simulink model "simulink_nivastyring"  (R2024b)
settings: Solver=VariableStepAuto  StartTime=0.0  StopTime=1000  RelTol=1e-6
undefined symbols (not defined in the file or in its folder): A_tank1, A_tank2, k, p
settings Model: Creator=serin  LastModifiedBy=seyon
settings SolverCC: ZeroCrossAlgorithm=Adaptive
settings DebuggingCC: IgnoredZcDiagnostic=none

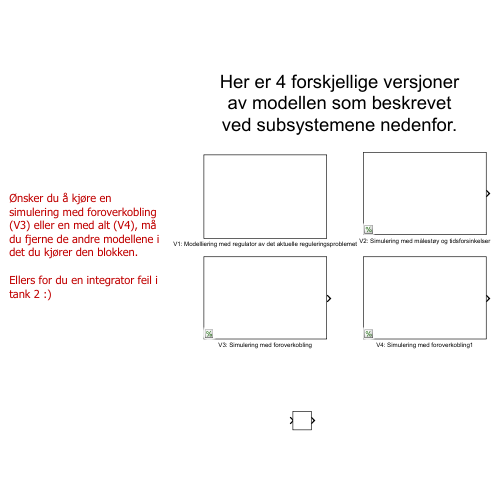
[thumbnail: Simulink's stored preview of the top-level diagram]
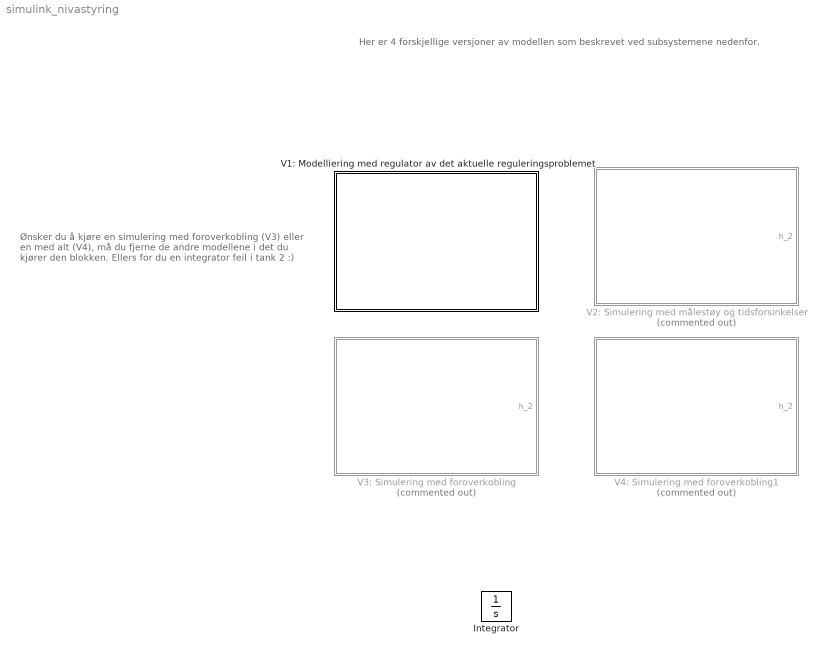
== system simulink_nivastyring ==
  note: Ønsker du å kjøre en simulering med foroverkobling (V3) eller en med alt (V4), må du fjerne de andre modellene i det du kjører den blokken.
      |
      | Ellers for du en integrator feil i tank 2 :)
  note: Her er 4 forskjellige versjoner av modellen som beskrevet ved subsystemene nedenfor.
  Integrator : Integrator
  V1: Modelliering med regulator av det aktuelle reguleringsproblemet : Subsystem
  V2: Simulering med målestøy og tidsforsinkelser : Subsystem  Commented=on
  V3: Simulering med foroverkobling : Subsystem  Commented=on
  V4: Simulering med foroverkobling1 : Subsystem  Commented=on

== system simulink_nivastyring/V1: Modelliering med regulator av det aktuelle reguleringsproblemet ==
  Scope : Scope  NumInputPorts=4
  Subsystem1 : Subsystem
  Subsystem2 : Subsystem
  Subsystem3 : Subsystem
  Subsystem4 : Subsystem
  wires:
  Subsystem1/1(h1) -> Scope/4  "tau = 0"
  Subsystem2/1(h1) -> Scope/1  "tau = 3"
  Subsystem3/1(h1) -> Scope/2  "tau = 6"
  Subsystem4/1(h1) -> Scope/3  "tau = 12"

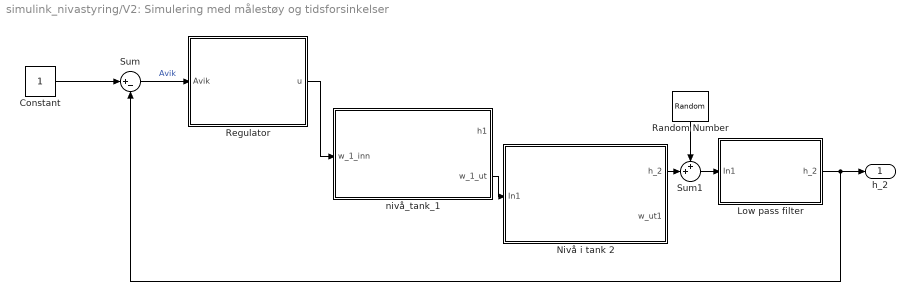
== system simulink_nivastyring/V2: Simulering med målestøy og tidsforsinkelser ==
  Constant : Constant
  Low pass filter : Subsystem
  Nivå i tank 2 : Subsystem
  Random Number : RandomNumber  Variance=0.001  Seed=23  SampleTime=1
  Regulator : Subsystem
  Sum : Sum  Inputs=|+-
  Sum1 : Sum  Inputs=++|
  nivå_tank_1 : Subsystem
  h_2 : Outport
  wires:
  Constant/1 -> Sum/1
  Nivå i tank 2/1(h_2) -> Sum1/2
  Sum1/1 -> Low pass filter/1(In1)
  Random Number/1 -> Sum1/1
  Low pass filter/1(h_2) -> h_2/1, Sum/2
  nivå_tank_1/2(w_1_ut) -> Nivå i tank 2/1(In1)
  Regulator/1(u) -> nivå_tank_1/1(w_1_inn)
  Sum/1 -> Regulator/1(Avik)  "Avik"

== system simulink_nivastyring/V3: Simulering med foroverkobling ==
  Constant : Constant
  Forstyrrelse1 : Subsystem
  Nivå i tank 2 : Subsystem
  Sum : Sum  Inputs=|+-
  Sum1 : Sum  Inputs=|++
  nivå_tank_1 : Subsystem
  regulator : Subsystem
  h_2 : Outport
  wires:
  Constant/1 -> Sum/1
  Nivå i tank 2/1(h_2) -> h_2/1, Sum/2
  nivå_tank_1/2(w_1_ut) -> Nivå i tank 2/1(In1)
  Sum/1 -> regulator/1(Avik)  "Avik"
  regulator/1(u) -> Sum1/1
  Forstyrrelse1/1(Out1) -> Sum1/2
  Sum1/1 -> nivå_tank_1/1(w_1_inn)

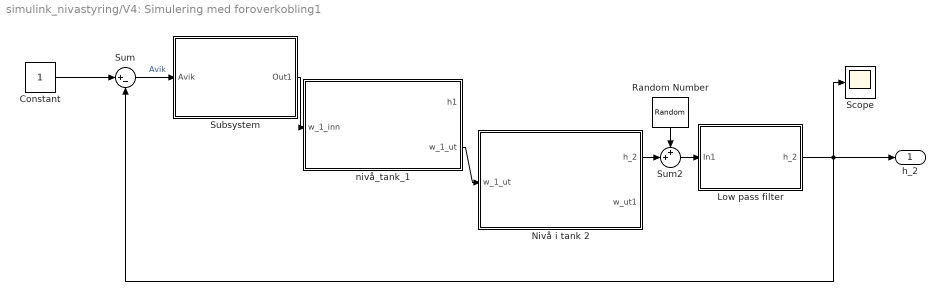
== system simulink_nivastyring/V4: Simulering med foroverkobling1 ==
  Constant : Constant
  Low pass filter : Subsystem
  Nivå i tank 2 : Subsystem
  Random Number : RandomNumber  Variance=0.001  Seed=23  SampleTime=1
  Scope : Scope
  Subsystem : Subsystem
  Sum : Sum  Inputs=|+-
  Sum2 : Sum  Inputs=++|
  nivå_tank_1 : Subsystem
  h_2 : Outport
  wires:
  Constant/1 -> Sum/1
  Nivå i tank 2/1(h_2) -> Sum2/2
  Random Number/1 -> Sum2/1
  nivå_tank_1/2(w_1_ut) -> Nivå i tank 2/1(w_1_ut)
  Sum2/1 -> Low pass filter/1(In1)
  Low pass filter/1(h_2) -> Scope/1, h_2/1, Sum/2
  Sum/1 -> Subsystem/1(Avik)  "Avik"
  Subsystem/1(Out1) -> nivå_tank_1/1(w_1_inn)

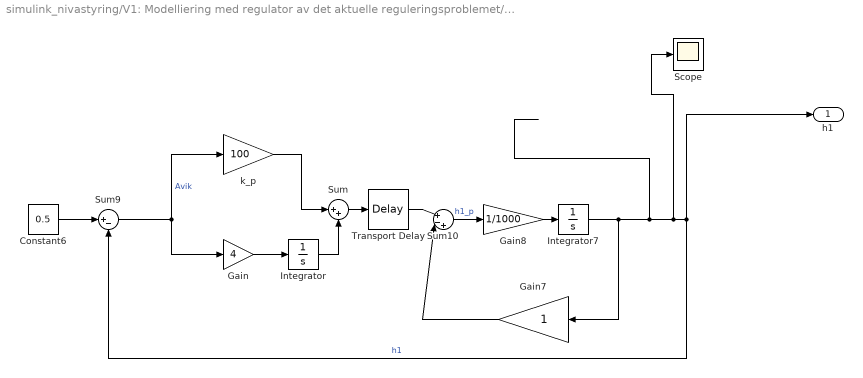
== system simulink_nivastyring/V1: Modelliering med regulator av det aktuelle reguleringsproblemet/Subsystem1 ==
  Constant6 : Constant  Value=0.5
  Gain : Gain  Gain=4
  Gain7 : Gain
  Gain8 : Gain  Gain=1/1000
  Integrator : Integrator
  Integrator7 : Integrator
  Scope : Scope
  Sum : Sum  Inputs=|++
  Sum10 : Sum  Inputs=|+-+
  Sum9 : Sum  Inputs=|+-
  Transport Delay : TransportDelay
  k_p : Gain  Gain=100
  h1 : Outport
  wires:
  Sum9/1 -> Gain/1, k_p/1  "Avik"
  Sum10/1 -> Gain8/1  "h1_p"
  Integrator7/1 -> Scope/1, h1/1, Sum9/2, Gain7/1  "h1"
  Gain7/1 -> Sum10/2
  Gain8/1 -> Integrator7/1
  Constant6/1 -> Sum9/1
  Gain/1 -> Integrator/1
  Integrator/1 -> Sum/2
  k_p/1 -> Sum/1
  Sum/1 -> Transport Delay/1
  Transport Delay/1 -> Sum10/1

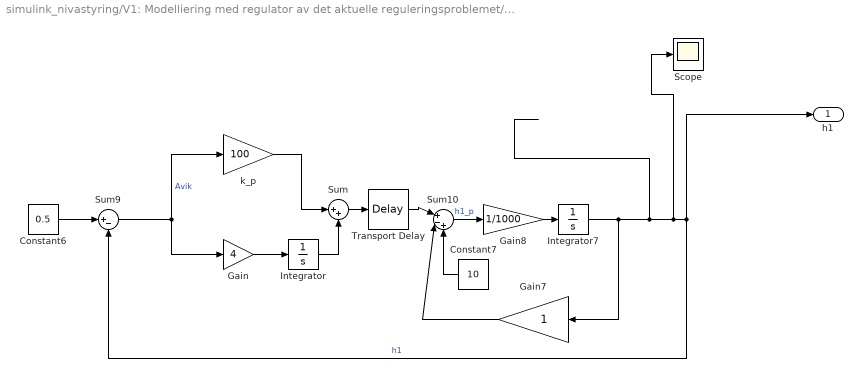
== system simulink_nivastyring/V1: Modelliering med regulator av det aktuelle reguleringsproblemet/Subsystem2 ==
  Constant6 : Constant  Value=0.5
  Constant7 : Constant  Value=10
  Gain : Gain  Gain=4
  Gain7 : Gain
  Gain8 : Gain  Gain=1/1000
  Integrator : Integrator
  Integrator7 : Integrator
  Scope : Scope
  Sum : Sum  Inputs=|++
  Sum10 : Sum  Inputs=|+-+
  Sum9 : Sum  Inputs=|+-
  Transport Delay : TransportDelay
  k_p : Gain  Gain=100
  h1 : Outport
  wires:
  Sum9/1 -> Gain/1, k_p/1  "Avik"
  Sum10/1 -> Gain8/1  "h1_p"
  Integrator7/1 -> Scope/1, h1/1, Sum9/2, Gain7/1  "h1"
  Gain7/1 -> Sum10/2
  Gain8/1 -> Integrator7/1
  Constant6/1 -> Sum9/1
  Constant7/1 -> Sum10/3
  Gain/1 -> Integrator/1
  Integrator/1 -> Sum/2
  k_p/1 -> Sum/1
  Sum/1 -> Transport Delay/1
  Transport Delay/1 -> Sum10/1

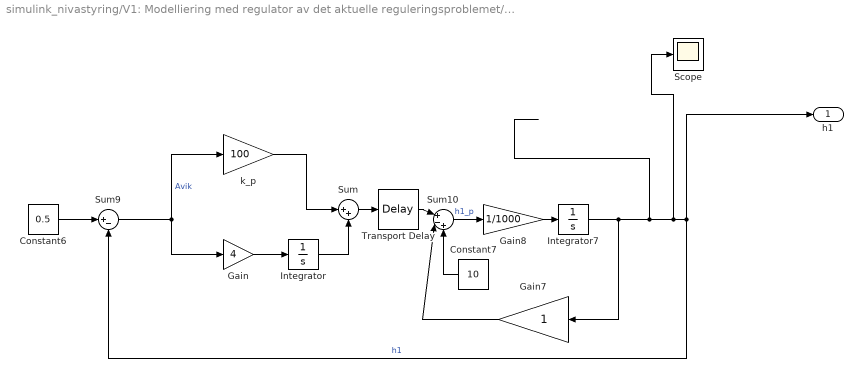
== system simulink_nivastyring/V1: Modelliering med regulator av det aktuelle reguleringsproblemet/Subsystem3 ==
  Constant6 : Constant  Value=0.5
  Constant7 : Constant  Value=10
  Gain : Gain  Gain=4
  Gain7 : Gain
  Gain8 : Gain  Gain=1/1000
  Integrator : Integrator
  Integrator7 : Integrator
  Scope : Scope
  Sum : Sum  Inputs=|++
  Sum10 : Sum  Inputs=|+-+
  Sum9 : Sum  Inputs=|+-
  Transport Delay : TransportDelay  DelayTime=6
  k_p : Gain  Gain=100
  h1 : Outport
  wires:
  Sum9/1 -> Gain/1, k_p/1  "Avik"
  Sum10/1 -> Gain8/1  "h1_p"
  Integrator7/1 -> Scope/1, h1/1, Sum9/2, Gain7/1  "h1"
  Gain7/1 -> Sum10/2
  Gain8/1 -> Integrator7/1
  Constant6/1 -> Sum9/1
  Constant7/1 -> Sum10/3
  Gain/1 -> Integrator/1
  Integrator/1 -> Sum/2
  k_p/1 -> Sum/1
  Sum/1 -> Transport Delay/1
  Transport Delay/1 -> Sum10/1

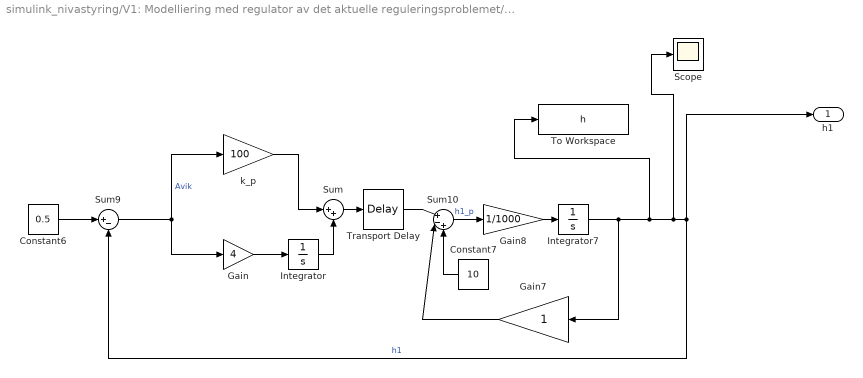
== system simulink_nivastyring/V1: Modelliering med regulator av det aktuelle reguleringsproblemet/Subsystem4 ==
  Constant6 : Constant  Value=0.5
  Constant7 : Constant  Value=10
  Gain : Gain  Gain=4
  Gain7 : Gain
  Gain8 : Gain  Gain=1/1000
  Integrator : Integrator
  Integrator7 : Integrator
  Scope : Scope
  Sum : Sum  Inputs=|++
  Sum10 : Sum  Inputs=|+-+
  Sum9 : Sum  Inputs=|+-
  To Workspace : ToWorkspace  VariableName=h  SaveFormat=Timeseries  SampleTime=-1
  Transport Delay : TransportDelay  DelayTime=12
  k_p : Gain  Gain=100
  h1 : Outport
  wires:
  Sum9/1 -> Gain/1, k_p/1  "Avik"
  Sum10/1 -> Gain8/1  "h1_p"
  Integrator7/1 -> To Workspace/1, Scope/1, h1/1, Sum9/2, Gain7/1  "h1"
  Gain7/1 -> Sum10/2
  Gain8/1 -> Integrator7/1
  Constant6/1 -> Sum9/1
  Constant7/1 -> Sum10/3
  Gain/1 -> Integrator/1
  Integrator/1 -> Sum/2
  k_p/1 -> Sum/1
  Sum/1 -> Transport Delay/1
  Transport Delay/1 -> Sum10/1

== system simulink_nivastyring/V2: Simulering med målestøy og tidsforsinkelser/Low pass filter ==
  In1 : Inport
  Gain : Gain  Gain=0.1
  Integrator : Integrator
  Sum2 : Sum  Inputs=|+-
  h_2 : Outport
  wires:
  Integrator/1 -> h_2/1, Sum2/2
  In1/1 -> Sum2/1
  Sum2/1 -> Gain/1
  Gain/1 -> Integrator/1

== system simulink_nivastyring/V2: Simulering med målestøy og tidsforsinkelser/Nivå i tank 2 ==
  In1 : Inport
  Gain5 : Gain  Gain=k
  Integrator3 : Integrator
  Square Root : Sqrt
  Sum4 : Sum  Inputs=+--
  verdi : Gain  Gain=1/(p*A_tank2)
  h_2 : Outport
  w_ut1 : Outport  Port=2
  wires:
  In1/1 -> Sum4/1
  Sum4/1 -> verdi/1
  Integrator3/1 -> h_2/1, Square Root/1
  Square Root/1 -> Gain5/1
  verdi/1 -> Integrator3/1
  Gain5/1 -> Sum4/2, w_ut1/1  "w_ut"

== system simulink_nivastyring/V2: Simulering med målestøy og tidsforsinkelser/Regulator ==
  Avik : Inport
  regulator : Subsystem  mask{kp=4.5, ki=0.01, wind_up=10}
  u : Outport
  wires:
  regulator/1(w_inn) -> u/1  "u"
  Avik/1 -> regulator/1(In1)

== system simulink_nivastyring/V2: Simulering med målestøy og tidsforsinkelser/nivå_tank_1 ==
  w_1_inn : Inport
  Gain2 : Gain  Gain=k
  Gain3 : Gain  Gain=1/(p*A_tank1)
  Integrator2 : Integrator
  Scope : Scope
  Square Root : Sqrt  OutputSignalType=real
  Sum : Sum  Inputs=|+-
  h1 : Outport
  w_1_ut : Outport  Port=2
  wires:
  Integrator2/1 -> Square Root/1, h1/1  "h1"
  Gain2/1 -> Scope/1, w_1_ut/1, Sum/2
  Sum/1 -> Gain3/1  "h1_p"
  Gain3/1 -> Integrator2/1
  w_1_inn/1 -> Sum/1
  Square Root/1 -> Gain2/1

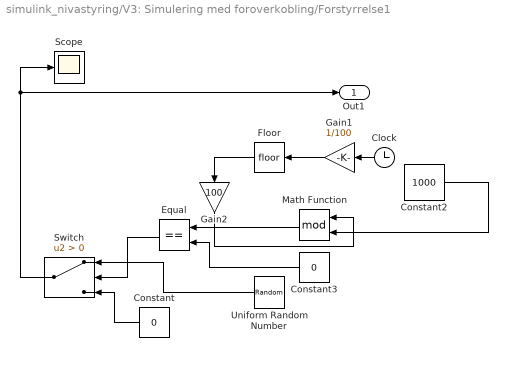
== system simulink_nivastyring/V3: Simulering med foroverkobling/Forstyrrelse1 ==
  Clock : Clock
  Constant : Constant  Value=0
  Constant2 : Constant  Value=1000
  Constant3 : Constant  Value=0
  Equal : RelationalOperator  Operator===  OutDataTypeStr=boolean  RndMeth=Simplest  InputSameDT=off
  Floor : Rounding
  Gain1 : Gain  Gain=1/100
  Gain2 : Gain  Gain=100
  Math Function : Math  Operator=mod
  Scope : Scope
  Switch : Switch  Criteria=u2 > Threshold  SaturateOnIntegerOverflow=off  InputSameDT=off
  Uniform Random Number : UniformRandomNumber  Minimum=0.08  Maximum=0.10  Seed=23  SampleTime=1
  Out1 : Outport
  wires:
  Gain2/1 -> Math Function/1
  Clock/1 -> Gain1/1
  Math Function/1 -> Equal/1
  Switch/1 -> Out1/1, Scope/1
  Constant2/1 -> Math Function/2
  Constant3/1 -> Equal/2
  Gain1/1 -> Floor/1
  Constant/1 -> Switch/3
  Equal/1 -> Switch/2
  Floor/1 -> Gain2/1
  Uniform Random Number/1 -> Switch/1

== system simulink_nivastyring/V3: Simulering med foroverkobling/Nivå i tank 2 ==
  In1 : Inport
  Gain5 : Gain  Gain=k
  Integrator3 : Integrator
  Square Root : Sqrt
  Sum4 : Sum  Inputs=+--
  verdi : Gain  Gain=1/(p*A_tank2)
  h_2 : Outport
  w_ut1 : Outport  Port=2
  wires:
  In1/1 -> Sum4/1
  Sum4/1 -> verdi/1
  Integrator3/1 -> Square Root/1, h_2/1
  Square Root/1 -> Gain5/1
  verdi/1 -> Integrator3/1
  Gain5/1 -> w_ut1/1, Sum4/2  "w_ut"

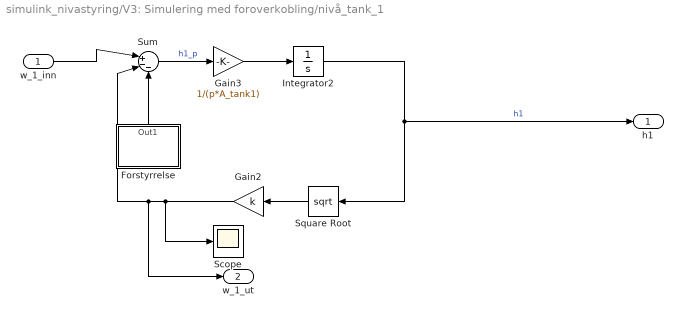
== system simulink_nivastyring/V3: Simulering med foroverkobling/nivå_tank_1 ==
  w_1_inn : Inport
  Forstyrrelse : Subsystem
  Gain2 : Gain  Gain=k
  Gain3 : Gain  Gain=1/(p*A_tank1)
  Integrator2 : Integrator
  Scope : Scope
  Square Root : Sqrt  OutputSignalType=real
  Sum : Sum  Inputs=|+--
  h1 : Outport
  w_1_ut : Outport  Port=2
  wires:
  Integrator2/1 -> Square Root/1, h1/1  "h1"
  Gain2/1 -> Sum/2, w_1_ut/1, Scope/1
  Sum/1 -> Gain3/1  "h1_p"
  Gain3/1 -> Integrator2/1
  w_1_inn/1 -> Sum/1
  Square Root/1 -> Gain2/1
  Forstyrrelse/1(Out1) -> Sum/3

== system simulink_nivastyring/V3: Simulering med foroverkobling/regulator ==
  Avik : Inport
  Rate Limiter : RateLimiter  FallingSlewLimit=-0.01  SampleTimeMode=inherited
  Saturation : Saturate  UpperLimit=4  LowerLimit=0
  ventilen : Subsystem  mask{kp=4.5, ki=0.01, wind_up=10}
  u : Outport
  wires:
  Saturation/1 -> Rate Limiter/1  "u"
  ventilen/1(w_inn) -> Saturation/1
  Avik/1 -> ventilen/1(In1)
  Rate Limiter/1 -> u/1

== system simulink_nivastyring/V4: Simulering med foroverkobling1/Low pass filter ==
  In1 : Inport
  Gain : Gain  Gain=0.1
  Integrator : Integrator
  Sum2 : Sum  Inputs=|+-
  h_2 : Outport
  wires:
  Integrator/1 -> h_2/1, Sum2/2
  In1/1 -> Sum2/1
  Sum2/1 -> Gain/1
  Gain/1 -> Integrator/1

== system simulink_nivastyring/V4: Simulering med foroverkobling1/Nivå i tank 2 ==
  w_1_ut : Inport
  Gain5 : Gain  Gain=k
  Integrator3 : Integrator
  Square Root : Sqrt
  Sum4 : Sum  Inputs=+--
  verdi : Gain  Gain=1/(p*A_tank2)
  h_2 : Outport
  w_ut1 : Outport  Port=2
  wires:
  w_1_ut/1 -> Sum4/1
  Sum4/1 -> verdi/1
  Integrator3/1 -> Square Root/1, h_2/1
  Square Root/1 -> Gain5/1
  verdi/1 -> Integrator3/1
  Gain5/1 -> w_ut1/1, Sum4/2  "w_ut"

== system simulink_nivastyring/V4: Simulering med foroverkobling1/Subsystem ==
  Avik : Inport
  Rate Limiter : RateLimiter  FallingSlewLimit=-0.01  SampleTimeMode=inherited
  Regulator : Subsystem  mask{kp=3, ki=0.0071, wind_up=10}
  Saturation : Saturate  UpperLimit=4  LowerLimit=0
  Sum1 : Sum  Inputs=|++
  Transport Delay : TransportDelay
  forstyrrelse_wv : Subsystem
  Out1 : Outport
  wires:
  Sum1/1 -> Rate Limiter/1  "u"
  Rate Limiter/1 -> Saturation/1
  forstyrrelse_wv/1(Out1) -> Sum1/2
  Transport Delay/1 -> Out1/1
  Regulator/1(w_inn) -> Sum1/1
  Saturation/1 -> Transport Delay/1  "u"
  Avik/1 -> Regulator/1(In1)

== system simulink_nivastyring/V4: Simulering med foroverkobling1/nivå_tank_1 ==
  w_1_inn : Inport
  Forstyrrelse : Subsystem
  Gain2 : Gain  Gain=k
  Gain3 : Gain  Gain=1/(p*A_tank1)
  Integrator2 : Integrator
  Square Root : Sqrt  OutputSignalType=real
  Sum : Sum  Inputs=|+--
  h1 : Outport
  w_1_ut : Outport  Port=2
  wires:
  Integrator2/1 -> Square Root/1, h1/1  "h1"
  Gain2/1 -> w_1_ut/1, Sum/2
  Sum/1 -> Gain3/1  "h1_p"
  Gain3/1 -> Integrator2/1
  w_1_inn/1 -> Sum/1
  Square Root/1 -> Gain2/1
  Forstyrrelse/1(Out1) -> Sum/3

== system simulink_nivastyring/V2: Simulering med målestøy og tidsforsinkelser/Regulator/regulator ==
  In1 : Inport
  Integrator : Integrator
  Rate Limiter : RateLimiter  FallingSlewLimit=-0.01  SampleTimeMode=inherited
  Saturation : Saturate  UpperLimit=4  LowerLimit=0
  Sum1 : Sum  Inputs=|+++
  k_i : Gain  Gain=ki
  k_p : Gain  Gain=kp
  w_inn : Outport
  wires:
  Integrator/1 -> Sum1/1
  In1/1 -> k_p/1, k_i/1
  k_p/1 -> Sum1/2
  Sum1/1 -> Saturation/1
  k_i/1 -> Integrator/1
  Saturation/1 -> Rate Limiter/1  "u"
  Rate Limiter/1 -> w_inn/1

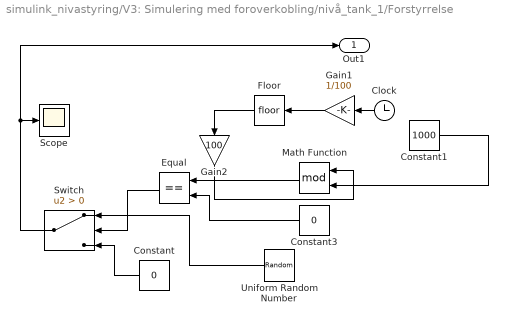
== system simulink_nivastyring/V3: Simulering med foroverkobling/nivå_tank_1/Forstyrrelse ==
  Clock : Clock
  Constant : Constant  Value=0
  Constant1 : Constant  Value=1000
  Constant3 : Constant  Value=0
  Equal : RelationalOperator  Operator===  OutDataTypeStr=boolean  RndMeth=Simplest  InputSameDT=off
  Floor : Rounding
  Gain1 : Gain  Gain=1/100
  Gain2 : Gain  Gain=100
  Math Function : Math  Operator=mod
  Scope : Scope
  Switch : Switch  Criteria=u2 > Threshold  SaturateOnIntegerOverflow=off  InputSameDT=off
  Uniform Random Number : UniformRandomNumber  Minimum=0.08  Maximum=0.10  Seed=23  SampleTime=1
  Out1 : Outport
  wires:
  Gain2/1 -> Math Function/1
  Clock/1 -> Gain1/1
  Math Function/1 -> Equal/1
  Switch/1 -> Scope/1, Out1/1
  Constant1/1 -> Math Function/2
  Constant3/1 -> Equal/2
  Gain1/1 -> Floor/1
  Constant/1 -> Switch/3
  Equal/1 -> Switch/2
  Floor/1 -> Gain2/1
  Uniform Random Number/1 -> Switch/1

== system simulink_nivastyring/V3: Simulering med foroverkobling/regulator/ventilen ==
  In1 : Inport
  Integrator : Integrator
  Sum1 : Sum  Inputs=++|
  k_i : Gain  Gain=ki
  k_p : Gain  Gain=kp
  w_inn : Outport
  wires:
  Integrator/1 -> Sum1/1
  In1/1 -> k_p/1, k_i/1
  k_p/1 -> Sum1/2
  k_i/1 -> Integrator/1
  Sum1/1 -> w_inn/1  "u"

== system simulink_nivastyring/V4: Simulering med foroverkobling1/Subsystem/Regulator ==
  In1 : Inport
  Integrator : Integrator
  Sum1 : Sum  Inputs=++|
  k_i : Gain  Gain=ki
  k_p : Gain  Gain=kp
  w_inn : Outport
  wires:
  Integrator/1 -> Sum1/1
  In1/1 -> k_p/1, k_i/1
  k_p/1 -> Sum1/2
  k_i/1 -> Integrator/1
  Sum1/1 -> w_inn/1  "u"

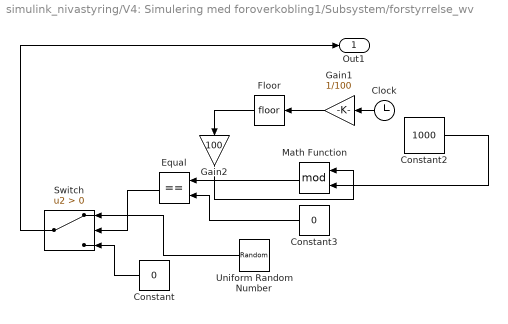
== system simulink_nivastyring/V4: Simulering med foroverkobling1/Subsystem/forstyrrelse_wv ==
  Clock : Clock
  Constant : Constant  Value=0
  Constant2 : Constant  Value=1000
  Constant3 : Constant  Value=0
  Equal : RelationalOperator  Operator===  OutDataTypeStr=boolean  RndMeth=Simplest  InputSameDT=off
  Floor : Rounding
  Gain1 : Gain  Gain=1/100
  Gain2 : Gain  Gain=100
  Math Function : Math  Operator=mod
  Switch : Switch  Criteria=u2 > Threshold  SaturateOnIntegerOverflow=off  InputSameDT=off
  Uniform Random Number : UniformRandomNumber  Minimum=0.1  Maximum=0.2  Seed=23  SampleTime=1
  Out1 : Outport
  wires:
  Gain2/1 -> Math Function/1
  Clock/1 -> Gain1/1
  Math Function/1 -> Equal/1
  Switch/1 -> Out1/1
  Constant2/1 -> Math Function/2
  Constant3/1 -> Equal/2
  Gain1/1 -> Floor/1
  Constant/1 -> Switch/3
  Equal/1 -> Switch/2
  Floor/1 -> Gain2/1
  Uniform Random Number/1 -> Switch/1

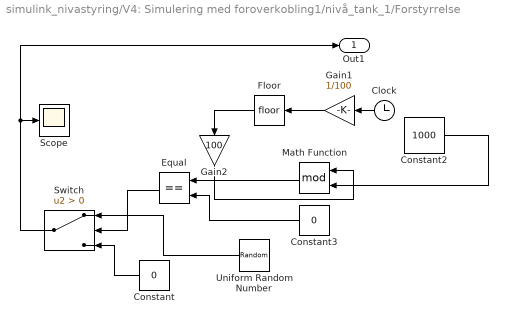
== system simulink_nivastyring/V4: Simulering med foroverkobling1/nivå_tank_1/Forstyrrelse ==
  Clock : Clock
  Constant : Constant  Value=0
  Constant2 : Constant  Value=1000
  Constant3 : Constant  Value=0
  Equal : RelationalOperator  Operator===  OutDataTypeStr=boolean  RndMeth=Simplest  InputSameDT=off
  Floor : Rounding
  Gain1 : Gain  Gain=1/100
  Gain2 : Gain  Gain=100
  Math Function : Math  Operator=mod
  Scope : Scope
  Switch : Switch  Criteria=u2 > Threshold  SaturateOnIntegerOverflow=off  InputSameDT=off
  Uniform Random Number : UniformRandomNumber  Minimum=0.18  Maximum=0.2  Seed=23  SampleTime=1
  Out1 : Outport
  wires:
  Gain2/1 -> Math Function/1
  Clock/1 -> Gain1/1
  Math Function/1 -> Equal/1
  Switch/1 -> Scope/1, Out1/1
  Constant2/1 -> Math Function/2
  Constant3/1 -> Equal/2
  Gain1/1 -> Floor/1
  Constant/1 -> Switch/3
  Equal/1 -> Switch/2
  Floor/1 -> Gain2/1
  Uniform Random Number/1 -> Switch/1
